simulink model "diffu_ctrl_sim"  (Simulink 8.3)
settings: Solver=ode45  StartTime=0.0  StopTime=10.0  FixedStep=0.025  RelTol=1e-3
values from neighbouring files (symbols this model uses):
  A = zeros((M-1)*(N-1))    [pre_process_Riesz_dh.m]
  DEXTRA = in(2*ND+3:end)    [distout.m]    (also in pre_process_Riesz_dh.m = [length(DPARA);DPARA(:)])
  fb = zeros([(M-1)*(N-1),1])    [pre_process_Riesz_dh.m]
  M = in(end-5)    [ctrldiscre.m]    (also in initialization1.m = 30; sensors.m = in(1))
  MEAN_SNOISE = 0    [initialization1.m]
  N = in(end-4)    [ctrldiscre.m]    (also in initialization1.m = 30; sensors.m = in(2))
  NA = in(2)    [actrl.m]    (also in actrl2.m; ades.m; controller.m = in(5*NS+2); ctrldiscre.m = in(1))
  ND = in(1)    [distout.m]    (also in initialization1.m = 1)
  NS = in(1)    [actrl.m]    (also in actrl2.m; ades.m; controller.m; initialization1.m = 841)
  PA0_1d = reshape(PA0, size_PA0(1)*size_PA0(2), 1)    [pre_process_Riesz_dh.m]
  PD0_1d = reshape(in(2:2*ND+1), ND, 2)    [distout.m]    (also in pre_process_Riesz_dh.m = reshape(PD0, size_PD0(1)*size_PD0(2), 1))
  PS0_1d = reshape(PS0, size_PS0(1)*size_PS0(2), 1)    [pre_process_Riesz_dh.m]
  SEED_SNOISE = 0:(M-1)*(N-1)-1    [pre_process_Riesz_dh.m]
  SNOISE_EXIST = 0    [initialization1.m]
  VAR_SNOISE = 0.04    [initialization1.m]
  VS0_1d = reshape(VS0, size_VS0(1)*size_VS0(2), 1)    [pre_process_Riesz_dh.m]
  ZERO_SNOISE = zeros((M-1)*(N-1),1)    [pre_process_Riesz_dh.m]
undefined symbols (not defined in the file or in its folder): u_0
settings Model: Creator=jsliang  LastModifiedBy=wayne  ExtModeAutoUpdateStatusClock=off
settings DataIOCC: SignalLoggingName=sigsOut
settings OptimizationCC: ExpressionDepthLimit=2147483647  InitFltsAndDblsToZero=on
settings DebuggingCC: SaveWithParameterizedLinksMsg=none  SignalResolutionControl=TryResolveAllWithWarning  SolverPrmCheckMsg=none  MultiTaskDSMMsg=warning  MultiTaskCondExecSysMsg=none  FcnCallInpInsideContextMsg=UseLocalSettings
settings HardwareCC: TargetUnknown=on
settings RTWCC: IncludeERTFirstTime=on
settings GRTTargetCC: TargetFcnLib=ansi_tfl_tmw.mat

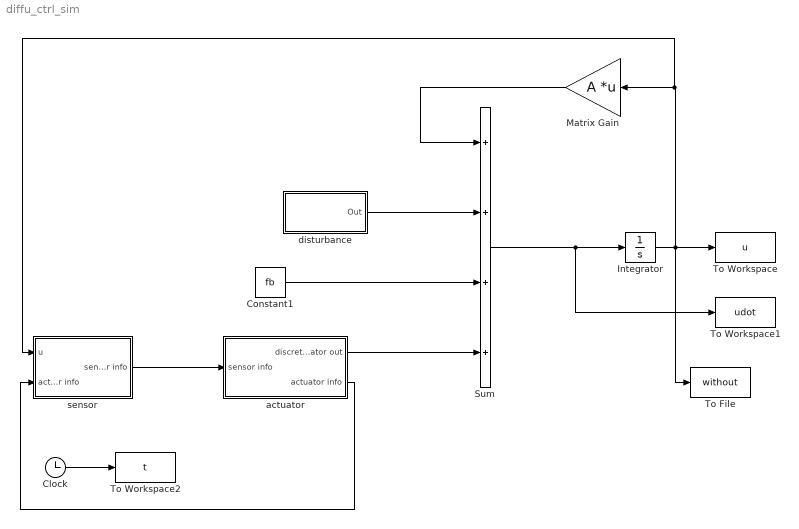
== system diffu_ctrl_sim ==
  Clock : Clock
  Constant1 : Constant  Value=fb
  Integrator : Integrator  InitialCondition=u_0
  Matrix Gain : Gain  Gain=A  Multiplication=Matrix(K*u) (u vector)  SaturateOnIntegerOverflow=on  OutDataTypeStr=Inherit: Same as input  ParamDataTypeStr=Inherit: Same as input
  Sum : Sum  Inputs=++++  SaturateOnIntegerOverflow=on
  To File : ToFile  Filename=without  MatrixName=without
  To Workspace : ToWorkspace  VariableName=u  SampleTime=-1
  To Workspace1 : ToWorkspace  VariableName=udot  SampleTime=-1
  To Workspace2 : ToWorkspace  VariableName=t  SampleTime=-1
  actuator : Subsystem
  "disturbance " : Subsystem
  "sensor " : Subsystem
  wires:
  Clock/1 -> To Workspace2/1
  Matrix Gain/1 -> Sum/1
  Sum/1 -> Integrator/1, To Workspace1/1
  Constant1/1 -> Sum/3
  actuator/1(discretized actuator out) -> Sum/4
  "sensor "/1(sensor info) -> actuator/1(sensor info)
  actuator/2(actuator info) -> "sensor "/2(actuator info)
  "disturbance "/1(Out) -> Sum/2
  Integrator/1 -> "sensor "/1(u), Matrix Gain/1, To Workspace/1, To File/1

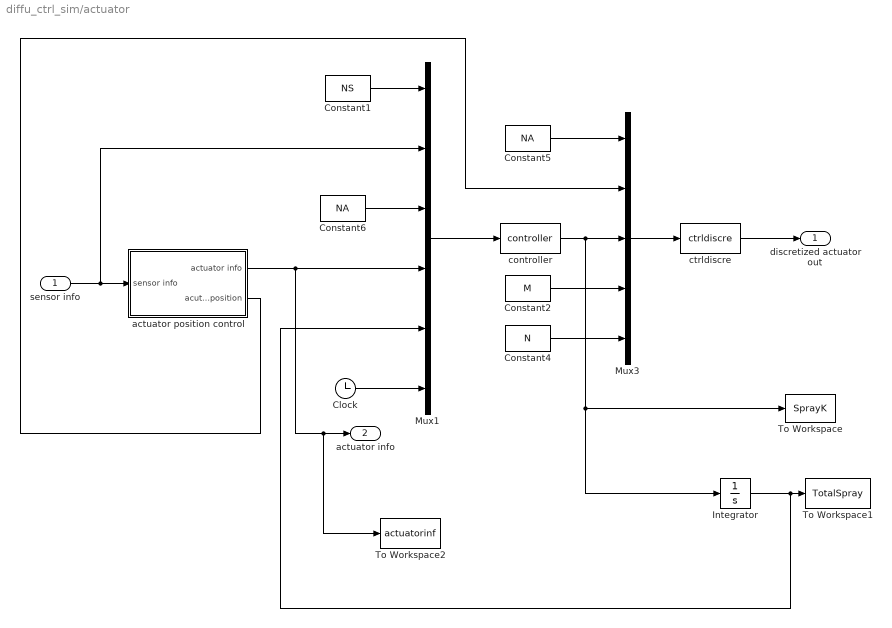
== system diffu_ctrl_sim/actuator ==
  sensor info : Inport
  Clock : Clock
  Constant1 : Constant  Value=NS
  Constant2 : Constant  Value=M
  Constant4 : Constant  Value=N
  Constant5 : Constant  Value=NA
  Constant6 : Constant  Value=NA
  Integrator : Integrator  InitialCondition=zeros(1,4)
  Mux1 : Mux  Inputs=6
  Mux3 : Mux  Inputs=5
  To Workspace : ToWorkspace  VariableName=SprayK  SampleTime=-1
  To Workspace1 : ToWorkspace  VariableName=TotalSpray  SampleTime=-1
  To Workspace2 : ToWorkspace  VariableName=actuatorinf  SampleTime=-1
  actuator position control : Subsystem
  controller : MATLABFcn  MATLABFcn=controller  OutputDimensions=NA  OutputSignalType=real
  ctrldiscre : MATLABFcn  MATLABFcn=ctrldiscre  OutputDimensions=(M-1)*(N-1)  OutputSignalType=real
  discretized actuator out : Outport
  actuator info : Outport  Port=2
  wires:
  Mux1/1 -> controller/1
  Constant1/1 -> Mux1/1
  Constant6/1 -> Mux1/3
  Clock/1 -> Mux1/6
  sensor info/1 -> actuator position control/1(sensor info), Mux1/2
  actuator position control/1(actuator info) -> Mux1/4, To Workspace2/1, actuator info/1
  Constant5/1 -> Mux3/1
  controller/1 -> Mux3/3, To Workspace/1, Integrator/1
  actuator position control/2(acutator position) -> Mux3/2
  Constant2/1 -> Mux3/4
  Constant4/1 -> Mux3/5
  Mux3/1 -> ctrldiscre/1
  ctrldiscre/1 -> discretized actuator out/1
  Integrator/1 -> To Workspace1/1, Mux1/5

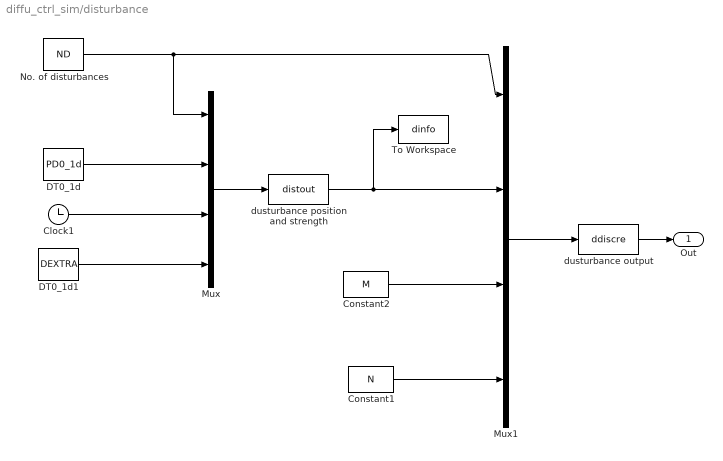
== system diffu_ctrl_sim/disturbance  ==
  Clock1 : Clock
  Constant1 : Constant  Value=N
  Constant2 : Constant  Value=M
  DT0_1d : Constant  Value=PD0_1d
  DT0_1d1 : Constant  Value=DEXTRA
  Mux : Mux
  Mux1 : Mux
  No. of disturbances : Constant  Value=ND
  To Workspace : ToWorkspace  VariableName=dinfo  SampleTime=-1
  dusturbance output : MATLABFcn  MATLABFcn=ddiscre  OutputDimensions=(M-1)*(N-1)  OutputSignalType=real
  dusturbance position and strength : MATLABFcn  MATLABFcn=distout  OutputDimensions=3*ND  OutputSignalType=real
  Out : Outport
  wires:
  Mux/1 -> dusturbance position and strength/1
  Mux1/1 -> dusturbance output/1
  dusturbance output/1 -> Out/1
  dusturbance position and strength/1 -> To Workspace/1, Mux1/2
  No. of disturbances/1 -> Mux/1, Mux1/1
  Constant2/1 -> Mux1/3
  Constant1/1 -> Mux1/4
  DT0_1d/1 -> Mux/2
  Clock1/1 -> Mux/3
  DT0_1d1/1 -> Mux/4

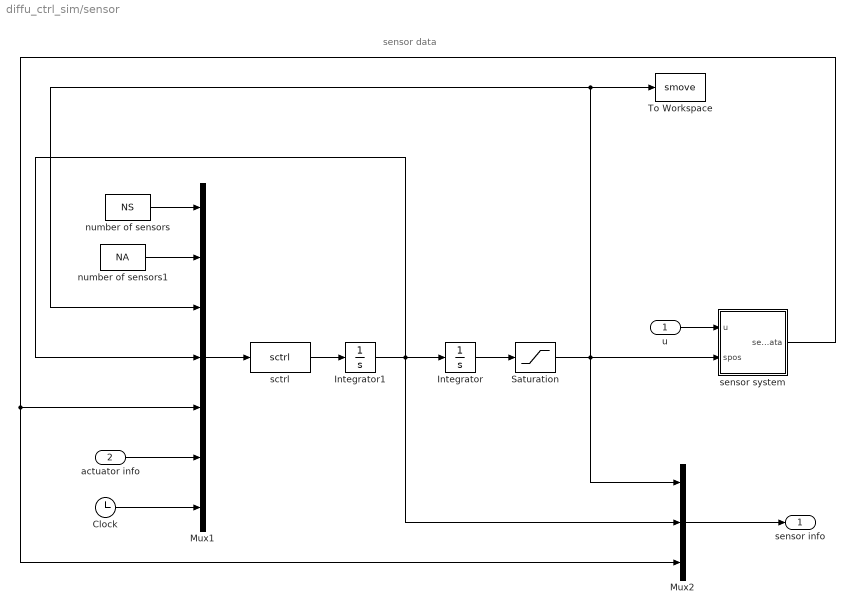
== system diffu_ctrl_sim/sensor  ==
  note: sensor data
  u : Inport
  actuator info : Inport  Port=2
  Clock : Clock
  Integrator : Integrator  InitialCondition=PS0_1d
  Integrator1 : Integrator  InitialCondition=VS0_1d
  Mux1 : Mux  Inputs=7
  Mux2 : Mux  Inputs=3
  Saturation : Saturate  UpperLimit=1  LowerLimit=0
  To Workspace : ToWorkspace  VariableName=smove  SampleTime=-1
  number of sensors : Constant  Value=NS
  number of sensors1 : Constant  Value=NA
  sctrl : MATLABFcn  MATLABFcn=sctrl  OutputDimensions=2*NS  OutputSignalType=real
  sensor system : Subsystem
  sensor info : Outport
  wires:
  sensor system/1(sensor data) -> Mux2/3, Mux1/5
  Integrator/1 -> Saturation/1
  Integrator1/1 -> Integrator/1, Mux2/2, Mux1/4
  sctrl/1 -> Integrator1/1
  Mux1/1 -> sctrl/1
  number of sensors/1 -> Mux1/1
  Mux2/1 -> sensor info/1
  number of sensors1/1 -> Mux1/2
  Clock/1 -> Mux1/7
  actuator info/1 -> Mux1/6
  u/1 -> sensor system/1(u)
  Saturation/1 -> Mux2/1, sensor system/2(spos), To Workspace/1, Mux1/3

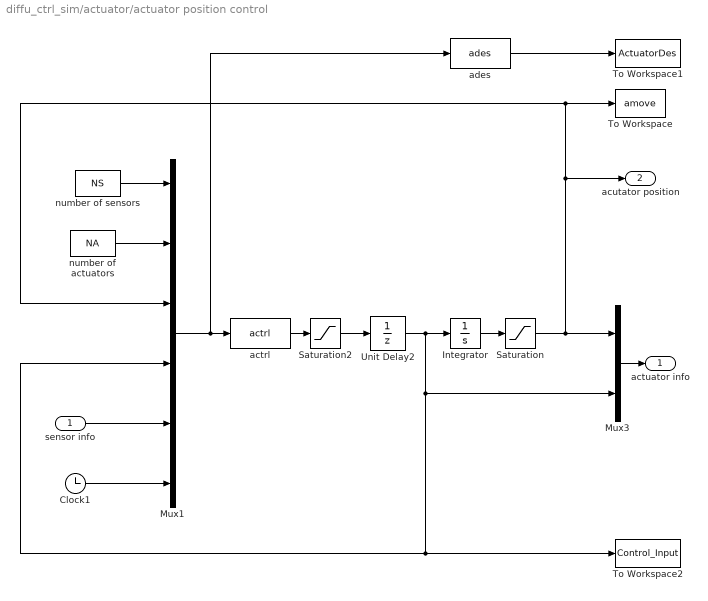
== system diffu_ctrl_sim/actuator/actuator position control ==
  sensor info : Inport
  Clock1 : Clock
  Integrator : Integrator  InitialCondition=PA0_1d
  Mux1 : Mux  Inputs=6
  Mux3 : Mux  Inputs=2
  Saturation : Saturate  UpperLimit=1  LowerLimit=0
  Saturation2 : Saturate  UpperLimit=0.1  LowerLimit=-0.1
  To Workspace : ToWorkspace  VariableName=amove  SampleTime=-1
  To Workspace1 : ToWorkspace  VariableName=ActuatorDes  SampleTime=-1
  To Workspace2 : ToWorkspace  VariableName=Control_Input  SampleTime=-1
  Unit Delay2 : UnitDelay  SampleTime=-1
  actrl : MATLABFcn  MATLABFcn=actrl  OutputDimensions=2*NA  OutputSignalType=real
  ades : MATLABFcn  MATLABFcn=ades  OutputDimensions=2*NA  OutputSignalType=real
  number of actuators : Constant  Value=NA
  number of sensors : Constant  Value=NS
  actuator info : Outport
  acutator position : Outport  Port=2
  wires:
  Integrator/1 -> Saturation/1
  Mux1/1 -> actrl/1, ades/1
  number of sensors/1 -> Mux1/1
  Mux3/1 -> actuator info/1
  number of actuators/1 -> Mux1/2
  sensor info/1 -> Mux1/5
  Clock1/1 -> Mux1/6
  Saturation/1 -> Mux3/1, To Workspace/1, Mux1/3, acutator position/1
  Saturation2/1 -> Unit Delay2/1
  ades/1 -> To Workspace1/1
  actrl/1 -> Saturation2/1
  Unit Delay2/1 -> Mux3/2, Mux1/4, To Workspace2/1, Integrator/1

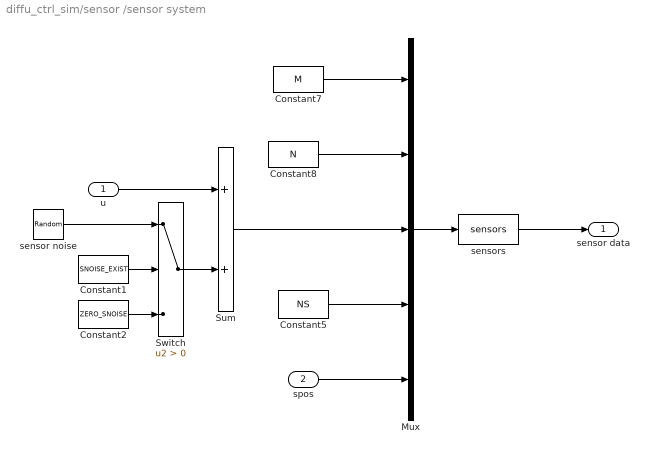
== system diffu_ctrl_sim/sensor /sensor system ==
  u : Inport
  spos : Inport  Port=2
  Constant1 : Constant  Value=SNOISE_EXIST
  Constant2 : Constant  Value=ZERO_SNOISE
  Constant5 : Constant  Value=NS
  Constant7 : Constant  Value=M
  Constant8 : Constant  Value=N
  Mux : Mux  Inputs=5
  Sum : Sum  SaturateOnIntegerOverflow=on
  Switch : Switch  Criteria=u2 > Threshold  SaturateOnIntegerOverflow=on
  sensor noise : RandomNumber  Mean=MEAN_SNOISE  Variance=VAR_SNOISE  Seed=SEED_SNOISE  SampleTime=0
  sensors : MATLABFcn  MATLABFcn=sensors  OutputDimensions=NS  OutputSignalType=real
  sensor data : Outport
  wires:
  Mux/1 -> sensors/1
  Constant7/1 -> Mux/1
  Constant8/1 -> Mux/2
  Constant5/1 -> Mux/4
  Sum/1 -> Mux/3
  u/1 -> Sum/1
  sensors/1 -> sensor data/1
  spos/1 -> Mux/5
  sensor noise/1 -> Switch/1
  Switch/1 -> Sum/2
  Constant1/1 -> Switch/2
  Constant2/1 -> Switch/3
